simulink model "orthosis_old"  (R2013a)
settings: Solver=FixedStepDiscrete  StartTime=0.0  StopTime=15  FixedStep=.1  RelTol=1e-3
undefined symbols (not defined in the file or in its folder): DiscIntNeverNeededParam
libraries: simulink x7
settings Model: xpc_rtwmakecfg_data=_xpccanac2pci_  BufferReuse=off  Creator=dholley  LastModifiedBy=dholley
settings SolverCC: AlgebraicLoopSolver=LineSearch
settings OptimizationCC: BlockReduction=off  OptimizeBlockIOStorage=off  BufferReuse=off  ExpressionFolding=off  LocalBlockOutputs=off
settings HardwareCC: ProdIntDivRoundTo=Zero  ProdEndianess=LittleEndian  ProdHWDeviceType=Generic->32-bit x86 compatible
settings RTWCC: SystemTargetFile=xpctarget.tlc  TemplateMakefile=xpc_default_tmf  Description=xPC Target  ProcessScript=xpctarget_make_rtw_hook  RTWCompilerOptimization=On
settings xpcTargetCC: TargetFcnLib=ansi_tfl_table_tmw.mat  CodeReplacementLibrary=XPC_BLAS  ParMdlRefBuildCompliant=on  ConcurrentExecutionCompliant=on  CombineSignalStateStructs=off  MATLABClassNameForMDSCustomization=xpcAperiodicCustomization  GRTInterface=on  GenerateAllocFcn=off  xPCTaskExecutionProfile=off  xPCRL32EventNumber=5000  xPCLoadParamSetFile=off  xPCConcurrentTasks=off  xPCEnableSFAnimation=off

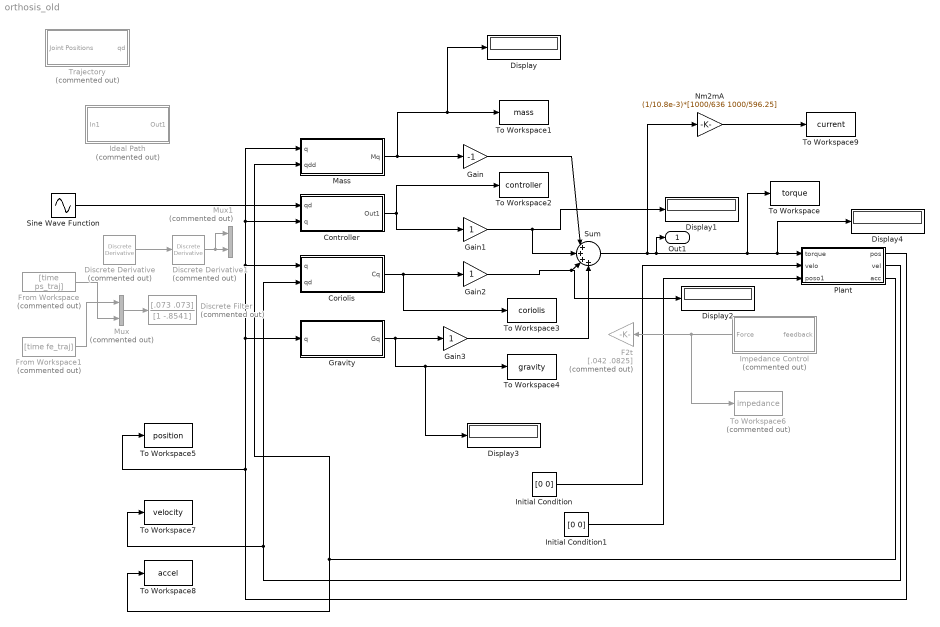
== system orthosis_old ==
  Controller : Subsystem  TreatAsAtomicUnit=on
      settings: RTWSystemCode=Inline
  Coriolis : Subsystem  TreatAsAtomicUnit=on
      settings: RTWSystemCode=Inline
  Discrete Derivative : simulink/Discrete/Discrete Derivative  Commented=on  gainval=1.0  ICPrevScaledInput=0.0  OutMin=[]  OutMax=[]  OutDataType=fixdt(1, 16)  OutScaling=2^-10  DoSatur=off
  Discrete Derivative1 : simulink/Discrete/Discrete Derivative  Commented=on  gainval=1.0  ICPrevScaledInput=0.0  OutMin=[]  OutMax=[]  OutDataType=fixdt(1, 16)  OutScaling=2^-10  DoSatur=off
  Discrete Filter : DiscreteFilter  Commented=on  Numerator=[.073 .073]  Denominator=[1 -.8541]  SampleTime=.001
  Display{,1..4} (5 alike) : Display
  F2t : Gain  Commented=on  Gain=[.042 .0825]
  From Workspace : FromWorkspace  Commented=on  VariableName=[time ps_traj]  SampleTime=0
  From Workspace1 : FromWorkspace  Commented=on  VariableName=[time fe_traj]  SampleTime=0
  Gain : Gain  Gain=-1
  Gain1 : Gain
  Gain2 : Gain
  Gain3 : Gain
  Gravity : Subsystem  TreatAsAtomicUnit=on
      settings: RTWSystemCode=Inline
  Ideal Path : Subsystem  Commented=on
  Impedance Control : Subsystem  Commented=on
  Initial Condition : Constant  Value=[0 0]
  Initial Condition1 : Constant  Value=[0 0]
  Mass : Subsystem  TreatAsAtomicUnit=on
      settings: RTWSystemCode=Inline
  Mux : Mux  Commented=on  Inputs=2
  Mux1 : Mux  Commented=on  Inputs=2
  Nm2mA : Gain  Gain=(1/10.8e-3)*[1000/636 1000/596.25]
  Plant : Subsystem  TreatAsAtomicUnit=on
      settings: MinAlgLoopOccurrences=on  RTWSystemCode=Inline
  Sine Wave Function : Sin  Amplitude=pi/4  Frequency=4
  Sum : Sum  Inputs=|++++
  To Workspace : ToWorkspace  VariableName=torque  SampleTime=-1  SaveFormat=Timeseries
  To Workspace1 : ToWorkspace  VariableName=mass  SampleTime=-1  SaveFormat=Timeseries
  To Workspace2 : ToWorkspace  VariableName=controller  SampleTime=-1  SaveFormat=Timeseries
  To Workspace3 : ToWorkspace  VariableName=coriolis  SampleTime=-1  SaveFormat=Timeseries
  To Workspace4 : ToWorkspace  VariableName=gravity  SampleTime=-1  SaveFormat=Timeseries
  To Workspace5 : ToWorkspace  VariableName=position  SampleTime=-1  SaveFormat=Timeseries
  To Workspace6 : ToWorkspace  Commented=on  VariableName=impedance  SampleTime=-1  SaveFormat=Timeseries
  To Workspace7 : ToWorkspace  VariableName=velocity  SampleTime=-1  SaveFormat=Timeseries
  To Workspace8 : ToWorkspace  VariableName=accel  SampleTime=-1  SaveFormat=Timeseries
  To Workspace9 : ToWorkspace  VariableName=current  SampleTime=-1  SaveFormat=Timeseries
  Trajectory : Subsystem  Commented=on
  Out1 : Outport
  wires:
  Mass/1(Mq) -> Gain/1, Display/1, To Workspace1/1
  Coriolis/1(Cq) -> To Workspace3/1, Gain2/1
  Gravity/1(Gq) -> Gain3/1, Display3/1, To Workspace4/1
  Controller/1(Out1) -> Gain1/1, To Workspace2/1
  Gain3/1 -> Sum/4
  Gain2/1 -> Display2/1, Sum/3
  Gain1/1 -> Display1/1, Sum/2
  Gain/1 -> Sum/1
  Plant/1(pos) -> Gravity/1(q), Controller/2(q), Mass/1(q), Coriolis/1(q), To Workspace5/1
  Initial Condition/1 -> Plant/2(velo)
  Initial Condition1/1 -> Plant/3(poso1)
  Plant/3(acc) -> Mass/2(qdd), To Workspace8/1
  Plant/2(vel) -> Coriolis/2(qd), To Workspace7/1
  Mux/1 -> Discrete Filter/1
  From Workspace/1 -> Mux/2
  From Workspace1/1 -> Mux/1
  Sum/1 -> Nm2mA/1, Out1/1, Display4/1, Plant/1(torque), To Workspace/1
  Sine Wave Function/1 -> Controller/1(qd)
  Impedance Control/1(Force) -> To Workspace6/1, F2t/1
  Discrete Derivative/1 -> Discrete Derivative1/1
  Discrete Derivative1/1 -> Mux1/1, Mux1/2
  Nm2mA/1 -> To Workspace9/1

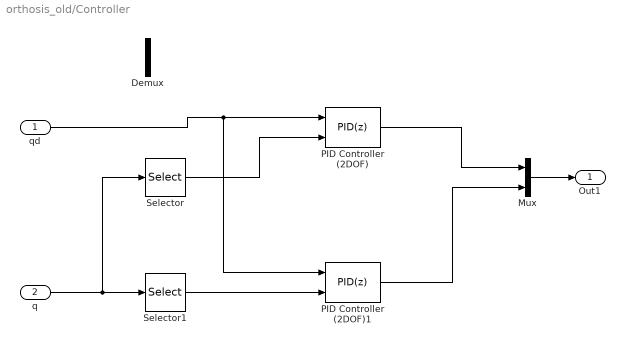
== system orthosis_old/Controller ==
  qd : Inport
  q : Inport  Port=2
  Demux : Demux  Outputs=2
  Mux : Mux  Inputs=2
  PID Controller (2DOF) : simulink/Continuous/PID Controller (2DOF)  Controller=PID  TimeDomain=Discrete-time  SampleTime=-1  IntegratorMethod=Forward Euler  FilterMethod=Forward Euler  Form=Parallel  P=0.000382424241826398  I=3.58199006661761e-06  D=0.00906317872058173  N=18.0350756688688  b=1  c=1  InitialConditionSource=internal  InitialConditionForIntegrator=0  InitialConditionForFilter=0  ExternalReset=none  LimitOutput=off  UpperSaturationLimit=inf  LowerSaturationLimit=-inf  LinearizeAsGain=on  AntiWindupMode=none  Kb=1  TrackingMode=off  Kt=1  PParamMin=[]  PParamMax=[]  IParamMin=[]  IParamMax=[]  DParamMin=[]  DParamMax=[]  NParamMin=[]  NParamMax=[]  bParamMin=[]  bParamMax=[]  cParamMin=[]  cParamMax=[]  KbParamMin=[]  KbParamMax=[]  KtParamMin=[]  KtParamMax=[]  POutMin=[]  POutMax=[]  IOutMin=[]  IOutMax=[]  DOutMin=[]  DOutMax=[]  NOutMin=[]  NOutMax=[]  bOutMin=[]  bOutMax=[]  cOutMin=[]  cOutMax=[]  KbOutMin=[]  KbOutMax=[]  KtOutMin=[]  KtOutMax=[]  IntegratorOutMin=[]  IntegratorOutMax=[]  FilterOutMin=[]  FilterOutMax=[]  SumOutMin=[]  SumOutMax=[]  Sum1OutMin=[]  Sum1OutMax=[]  Sum2OutMin=[]  Sum2OutMax=[]  Sum3OutMin=[]  Sum3OutMax=[]  SumI1OutMin=[]  SumI1OutMax=[]  SumI2OutMin=[]  SumI2OutMax=[]  SumI3OutMin=[]  SumI3OutMax=[]  SumDOutMin=[]  SumDOutMax=[]  SaturationOutMin=[]  SaturationOutMax=[]  IntegratorContinuousStateAttributes=''  IntegratorStateMustResolveToSignalObject=off  IntegratorRTWStateStorageClass=Auto  FilterContinuousStateAttributes=''  FilterStateMustResolveToSignalObject=off  FilterRTWStateStorageClass=Auto
  PID Controller (2DOF)1 : simulink/Continuous/PID Controller (2DOF)  Controller=PID  TimeDomain=Discrete-time  SampleTime=-1  IntegratorMethod=Forward Euler  FilterMethod=Forward Euler  Form=Parallel  P=5  I=10  D=2  N=200  b=1  c=1  InitialConditionSource=internal  InitialConditionForIntegrator=0  InitialConditionForFilter=0  ExternalReset=none  LimitOutput=off  UpperSaturationLimit=inf  LowerSaturationLimit=-inf  LinearizeAsGain=on  AntiWindupMode=none  Kb=1  TrackingMode=off  Kt=1  PParamMin=[]  PParamMax=[]  IParamMin=[]  IParamMax=[]  DParamMin=[]  DParamMax=[]  NParamMin=[]  NParamMax=[]  bParamMin=[]  bParamMax=[]  cParamMin=[]  cParamMax=[]  KbParamMin=[]  KbParamMax=[]  KtParamMin=[]  KtParamMax=[]  POutMin=[]  POutMax=[]  IOutMin=[]  IOutMax=[]  DOutMin=[]  DOutMax=[]  NOutMin=[]  NOutMax=[]  bOutMin=[]  bOutMax=[]  cOutMin=[]  cOutMax=[]  KbOutMin=[]  KbOutMax=[]  KtOutMin=[]  KtOutMax=[]  IntegratorOutMin=[]  IntegratorOutMax=[]  FilterOutMin=[]  FilterOutMax=[]  SumOutMin=[]  SumOutMax=[]  Sum1OutMin=[]  Sum1OutMax=[]  Sum2OutMin=[]  Sum2OutMax=[]  Sum3OutMin=[]  Sum3OutMax=[]  SumI1OutMin=[]  SumI1OutMax=[]  SumI2OutMin=[]  SumI2OutMax=[]  SumI3OutMin=[]  SumI3OutMax=[]  SumDOutMin=[]  SumDOutMax=[]  SaturationOutMin=[]  SaturationOutMax=[]  IntegratorContinuousStateAttributes=''  IntegratorStateMustResolveToSignalObject=off  IntegratorRTWStateStorageClass=Auto  FilterContinuousStateAttributes=''  FilterStateMustResolveToSignalObject=off  FilterRTWStateStorageClass=Auto
  Selector : Selector  InputPortWidth=2  IndexOptions=Index vector (dialog)  Indices=[1]  OutputSizes=1
  Selector1 : Selector  InputPortWidth=2  IndexOptions=Index vector (dialog)  Indices=[2]  OutputSizes=1
  Out1 : Outport
  wires:
  q/1 -> Selector/1, Selector1/1
  Selector/1 -> PID Controller (2DOF)/2
  Selector1/1 -> PID Controller (2DOF)1/2
  Mux/1 -> Out1/1
  qd/1 -> PID Controller (2DOF)1/1, PID Controller (2DOF)/1
  PID Controller (2DOF)/1 -> Mux/1
  PID Controller (2DOF)1/1 -> Mux/2

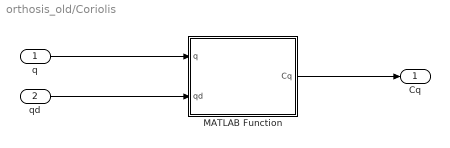
== system orthosis_old/Coriolis ==
  q : Inport
  qd : Inport  Port=2
  MATLAB Function : MATLAB Function  TreatAsAtomicUnit=on
  Cq : Outport
  wires:
  q/1 -> MATLAB Function/1(q)
  MATLAB Function/1(Cq) -> Cq/1
  qd/1 -> MATLAB Function/2(qd)

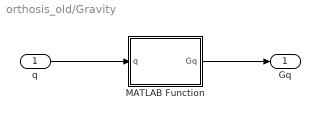
== system orthosis_old/Gravity ==
  q : Inport
  MATLAB Function : MATLAB Function  TreatAsAtomicUnit=on
  Gq : Outport
  wires:
  q/1 -> MATLAB Function/1(q)
  MATLAB Function/1(Gq) -> Gq/1

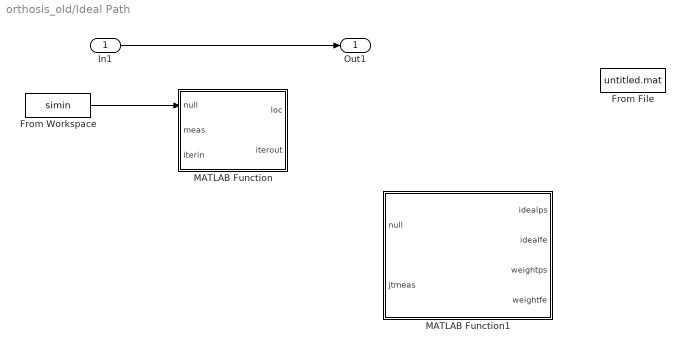
== system orthosis_old/Ideal Path ==
  In1 : Inport
  From Workspace : FromWorkspace  VariableName=simin  SampleTime=0
  From File : FromFile  SampleTime=0
  MATLAB Function : MATLAB Function  TreatAsAtomicUnit=on
  MATLAB Function1 : MATLAB Function  TreatAsAtomicUnit=on
  Out1 : Outport
  wires:
  In1/1 -> Out1/1
  From Workspace/1 -> MATLAB Function/1(null)

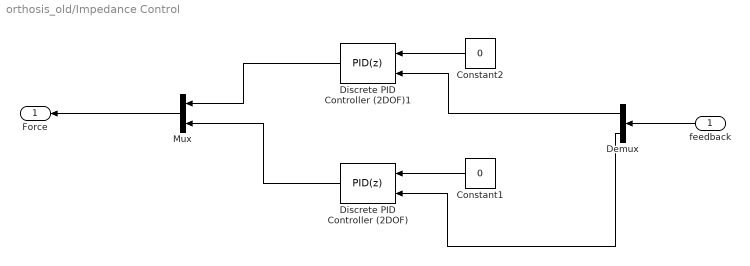
== system orthosis_old/Impedance Control ==
  feedback : Inport
  Constant1 : Constant  Value=0
  Constant2 : Constant  Value=0
  Demux : Demux  Outputs=2
  Discrete PID Controller (2DOF) : simulink/Continuous/PID Controller (2DOF)  Controller=PID  TimeDomain=Discrete-time  SampleTime=.001  IntegratorMethod=Forward Euler  FilterMethod=Forward Euler  Form=Parallel  P=10  I=1  D=0  N=100  b=1  c=1  InitialConditionSource=internal  InitialConditionForIntegrator=0  InitialConditionForFilter=0  ExternalReset=none  LimitOutput=off  UpperSaturationLimit=inf  LowerSaturationLimit=-inf  LinearizeAsGain=off  AntiWindupMode=none  Kb=1  TrackingMode=off  Kt=1  PParamMin=[]  PParamMax=[]  IParamMin=[]  IParamMax=[]  DParamMin=[]  DParamMax=[]  NParamMin=[]  NParamMax=[]  bParamMin=[]  bParamMax=[]  cParamMin=[]  cParamMax=[]  KbParamMin=[]  KbParamMax=[]  KtParamMin=[]  KtParamMax=[]  POutMin=[]  POutMax=[]  IOutMin=[]  IOutMax=[]  DOutMin=[]  DOutMax=[]  NOutMin=[]  NOutMax=[]  bOutMin=[]  bOutMax=[]  cOutMin=[]  cOutMax=[]  KbOutMin=[]  KbOutMax=[]  KtOutMin=[]  KtOutMax=[]  IntegratorOutMin=[]  IntegratorOutMax=[]  FilterOutMin=[]  FilterOutMax=[]  SumOutMin=[]  SumOutMax=[]  Sum1OutMin=[]  Sum1OutMax=[]  Sum2OutMin=[]  Sum2OutMax=[]  Sum3OutMin=[]  Sum3OutMax=[]  SumI1OutMin=[]  SumI1OutMax=[]  SumI2OutMin=[]  SumI2OutMax=[]  SumI3OutMin=[]  SumI3OutMax=[]  SumDOutMin=[]  SumDOutMax=[]  SaturationOutMin=[]  SaturationOutMax=[]  IntegratorContinuousStateAttributes=''  IntegratorStateMustResolveToSignalObject=off  IntegratorRTWStateStorageClass=Auto  FilterContinuousStateAttributes=''  FilterStateMustResolveToSignalObject=off  FilterRTWStateStorageClass=Auto
  Discrete PID Controller (2DOF)1 : simulink/Continuous/PID Controller (2DOF)  Controller=PID  TimeDomain=Discrete-time  SampleTime=.001  IntegratorMethod=Forward Euler  FilterMethod=Forward Euler  Form=Parallel  P=10  I=10  D=0  N=100  b=1  c=1  InitialConditionSource=internal  InitialConditionForIntegrator=0  InitialConditionForFilter=0  ExternalReset=none  LimitOutput=off  UpperSaturationLimit=inf  LowerSaturationLimit=-inf  LinearizeAsGain=off  AntiWindupMode=none  Kb=1  TrackingMode=off  Kt=1  PParamMin=[]  PParamMax=[]  IParamMin=[]  IParamMax=[]  DParamMin=[]  DParamMax=[]  NParamMin=[]  NParamMax=[]  bParamMin=[]  bParamMax=[]  cParamMin=[]  cParamMax=[]  KbParamMin=[]  KbParamMax=[]  KtParamMin=[]  KtParamMax=[]  POutMin=[]  POutMax=[]  IOutMin=[]  IOutMax=[]  DOutMin=[]  DOutMax=[]  NOutMin=[]  NOutMax=[]  bOutMin=[]  bOutMax=[]  cOutMin=[]  cOutMax=[]  KbOutMin=[]  KbOutMax=[]  KtOutMin=[]  KtOutMax=[]  IntegratorOutMin=[]  IntegratorOutMax=[]  FilterOutMin=[]  FilterOutMax=[]  SumOutMin=[]  SumOutMax=[]  Sum1OutMin=[]  Sum1OutMax=[]  Sum2OutMin=[]  Sum2OutMax=[]  Sum3OutMin=[]  Sum3OutMax=[]  SumI1OutMin=[]  SumI1OutMax=[]  SumI2OutMin=[]  SumI2OutMax=[]  SumI3OutMin=[]  SumI3OutMax=[]  SumDOutMin=[]  SumDOutMax=[]  SaturationOutMin=[]  SaturationOutMax=[]  IntegratorContinuousStateAttributes=''  IntegratorStateMustResolveToSignalObject=off  IntegratorRTWStateStorageClass=Auto  FilterContinuousStateAttributes=''  FilterStateMustResolveToSignalObject=off  FilterRTWStateStorageClass=Auto
  Mux : Mux  Inputs=2
  Force : Outport
  wires:
  Constant1/1 -> Discrete PID Controller (2DOF)/1
  Constant2/1 -> Discrete PID Controller (2DOF)1/1
  Discrete PID Controller (2DOF)1/1 -> Mux/1
  Discrete PID Controller (2DOF)/1 -> Mux/2
  Mux/1 -> Force/1
  feedback/1 -> Demux/1
  Demux/2 -> Discrete PID Controller (2DOF)/2
  Demux/1 -> Discrete PID Controller (2DOF)1/2

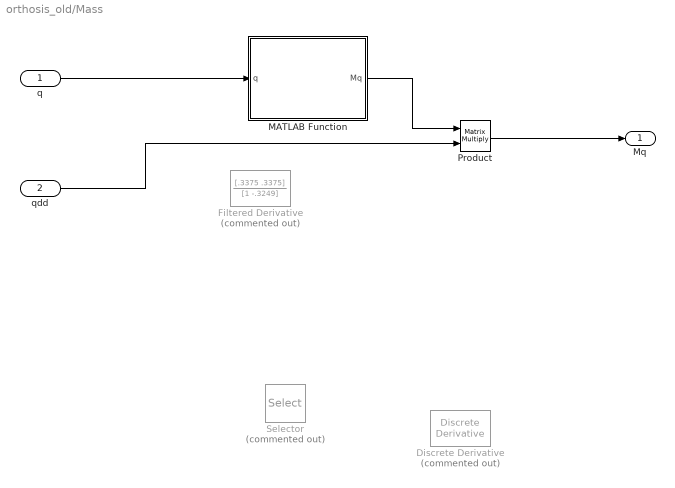
== system orthosis_old/Mass ==
  q : Inport
  qdd : Inport  Port=2
  Discrete Derivative : simulink/Discrete/Discrete Derivative  Commented=on  gainval=.1  ICPrevScaledInput=0.0  OutMin=[]  OutMax=[]  OutDataType=fixdt(1, 16)  OutScaling=2^-10  DoSatur=off
  Filtered Derivative : DiscreteFilter  Commented=on  Numerator=[.3375 .3375]  Denominator=[1 -.3249]  SampleTime=.1
  MATLAB Function : MATLAB Function  TreatAsAtomicUnit=on
  Product : Product  Multiplication=Matrix(*)  RndMeth=Zero
  Selector : Selector  Commented=on  InputPortWidth=4  IndexOptions=Index vector (dialog)  Indices=[3:4]  OutputSizes=1
  Mq : Outport
  wires:
  q/1 -> MATLAB Function/1(q)
  MATLAB Function/1(Mq) -> Product/1
  Product/1 -> Mq/1
  qdd/1 -> Product/2

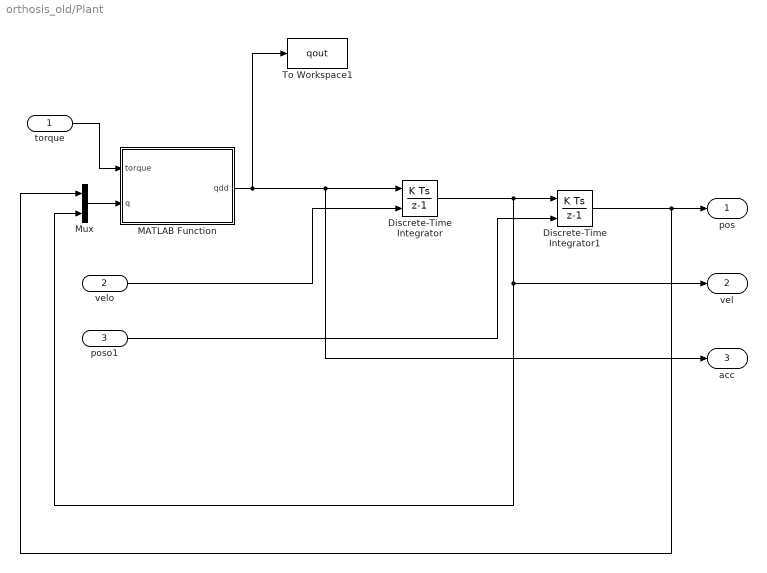
== system orthosis_old/Plant ==
  torque : Inport
  velo : Inport  Port=2
  poso1 : Inport  Port=3
  Discrete-Time Integrator : DiscreteIntegrator  gainval=1  InitialConditionSource=external  SampleTime=-1  ICPrevOutput=DiscIntNeverNeededParam  ICPrevScaledInput=DiscIntNeverNeededParam
  Discrete-Time Integrator1 : DiscreteIntegrator  gainval=1  InitialConditionSource=external  SampleTime=-1  ICPrevOutput=DiscIntNeverNeededParam  ICPrevScaledInput=DiscIntNeverNeededParam
  MATLAB Function : MATLAB Function  TreatAsAtomicUnit=on
  Mux : Mux  Inputs=2
  To Workspace1 : ToWorkspace  VariableName=qout  SampleTime=-1  SaveFormat=Timeseries
  pos : Outport
  vel : Outport  Port=2
  acc : Outport  Port=3
  wires:
  torque/1 -> MATLAB Function/1(torque)
  MATLAB Function/1(qdd) -> acc/1, Discrete-Time Integrator/1, To Workspace1/1
  velo/1 -> Discrete-Time Integrator/2
  Discrete-Time Integrator1/1 -> Mux/1, pos/1
  Discrete-Time Integrator/1 -> vel/1, Mux/2, Discrete-Time Integrator1/1
  poso1/1 -> Discrete-Time Integrator1/2
  Mux/1 -> MATLAB Function/2(q)

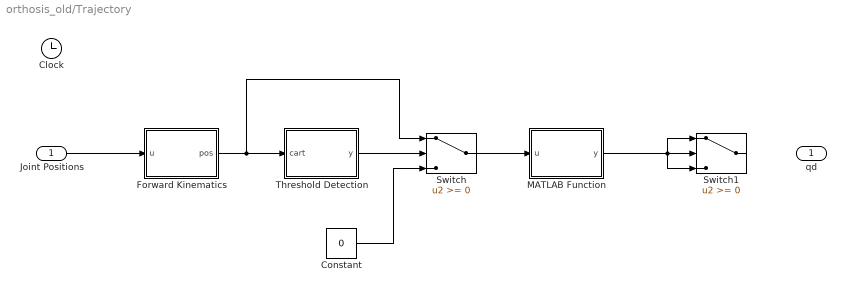
== system orthosis_old/Trajectory ==
  Joint Positions : Inport
  Clock : Clock
  Constant : Constant  Value=0
  Forward Kinematics : MATLAB Function  TreatAsAtomicUnit=on
  MATLAB Function : MATLAB Function  TreatAsAtomicUnit=on
  Switch : Switch
  Switch1 : Switch
  Threshold Detection : MATLAB Function  TreatAsAtomicUnit=on
  qd : Outport
  wires:
  Joint Positions/1 -> Forward Kinematics/1(u)
  Forward Kinematics/1(pos) -> Switch/1, Threshold Detection/1(cart)
  Threshold Detection/1(y) -> Switch/2
  Constant/1 -> Switch/3
  Switch/1 -> MATLAB Function/1(u)
  MATLAB Function/1(y) -> Switch1/3, Switch1/1, Switch1/2

== matlab function orthosis_old/Coriolis/MATLAB Function ==
  data: q input; Cq output; qd input
function Cq = Coriolis(q,qd)
%#codegen

weight=(85.4');%kg
hand_length=(.189);%m
hand_width=(.084);%m

s7=sin(q(2));
c7=cos(q(2));
a7cm=-.00458;
d7cm=-.00285;
a6=.03952;
m7=.2256; %kg

hand_xcom=0;
hand_ycom=-hand_length*.468;
hand_zcom=hand_width/2;
hand_mass=weight*.00575;

com7=[a7cm;-.03363;d7cm]*m7 + [hand_xcom;hand_ycom;hand_zcom]*hand_mass/(m7 + hand_mass);

%Centrifugal
c112=-m7*com7(1)^2*s7*c7;
C1C2=[0 0;c112 0];

%Coriolis
c121=-m7*com7(1)^2*s7*c7;
c122=m7*com7(1)*com7(3)*c7;
C22=[c121;c122];

Cq=C22*(qd(1)*qd(2)) + C1C2*[qd(1)^2;qd(2)^2];

== matlab function orthosis_old/Mass/MATLAB Function ==
  data: q input; Mq output
function Mq  = massmatrix(q)

%%Input Metrics
height=(1.776);%m
weight=(85.4);%kg
hand_length=(.189);%m
hand_width=(.084);%m
hand_thick=(.028);%m

% s1=sind(q(1));
% c1=cosd(q(1));
% s2=sind(q(2));
% c2=cosd(q(2));
% s4=sind(q(4));
% c4=cosd(q(4));
% s5=sind(q(5));
% c5=cosd(q(5));
s6=sin(q(1));
c6=cos(q(1));
s7=sin(q(2));
c7=cos(q(2));

m6=.4242; %kg
m7=.2256; %kg

%in m
a6cm=.02382;
d6cm=.04397;
a7cm=-.00458;
d7cm=-.00285;
d6=.06708;
a6=.03952;
a5=.12051;
d4=.04586;
a2=.37546;
d1=.33655;

%Forearm Inertia
forearm_length=height*.1585;
forearm_mass=weight*.016;
forearm_volume=forearm_mass/1062;
forearm_radius=sqrt(forearm_volume/(pi*forearm_length));

arm_zcom=d6-(forearm_length*.568);
arm_xcom=a6-forearm_radius;
arm_ycom=0;


kx_forearm=forearm_radius*.276;
ky_forearm=forearm_radius*.265;
kz_forearm=forearm_length*.121;
Ixx_forearm=forearm_mass*kx_forearm^2 + forearm_mass*arm_zcom^2;
Iyy_forearm=forearm_mass*ky_forearm^2 + forearm_mass*(arm_xcom^2 + arm_zcom^2);
Izz_forearm=forearm_mass*kz_forearm^2 + forearm_mass*arm_xcom^2;
Ixy_forearm=0;
Ixz_forearm=forearm_mass*arm_xcom*arm_zcom;
Iyz_forearm=0;

I_forearm=[Ixx_forearm,-Ixy_forearm,-Ixz_forearm;-Ixy_forearm,Iyy_forearm,-Iyz_forearm;-Ixz_forearm,-Iyz_forearm,Izz_forearm];

%Hand Inertia
hand_xcom=0;
hand_ycom=-hand_length*.468;
hand_zcom=hand_width/2;
hand_mass=weight*.00575;

kx_hand=hand_thick*.235;
ky_hand=hand_length*.184;
kz_hand=hand_width*.288;
Ixx_hand=hand_mass*kx_hand^2 + hand_mass*(hand_ycom^2 + hand_zcom^2);
Iyy_hand=hand_mass*ky_hand^2 + hand_mass*hand_zcom^2;
Izz_hand=hand_mass*kz_hand^2 + hand_mass*hand_ycom^2;
Ixy_hand=0;
Ixz_hand=0;
Iyz_hand=hand_mass*hand_ycom*hand_zcom;

I_hand=[Ixx_hand,-Ixy_hand,-Ixz_hand;-Ixy_hand,Iyy_hand,-Iyz_hand;-Ixz_hand,-Iyz_hand,Izz_hand];


I6=[2.259e-3 -7.049e-5 -9.252e-5;-7.049e-5 2.091e-3 -4.603e-4;-9.252e-5 -4.603e-4 8.911e-4];
I7=[7.022e-4 8.207e-5 -2.535e-5;8.207e-5 1.675e-4 -1.046e-4;-2.535e-5 -1.046e-4 6.273e-4];

%Forward Kinematics for Positioning
% x=-a5*c1*s2*c5 - a5*s5*(s1*c4 - c1*c2*s4) - d4*c1*s2 + d3*c1*c2 + a2*c1*c2;
% y=-a5*s1*s2*c5 + a5*s5*(c1*c4 + s1*c2*c4) - d4*s1*s2 + d3*s1*c2 + a2*s1*c2;
% z=-a5*c2*c5 - a5*s2*s4*s5 - d4*c2 - d3*s2 - a2*s2 + d1;

%Modified Center of Mass Location
com6=[a6cm;-.01547;d6cm]*m6 + [arm_xcom;arm_ycom;arm_zcom]*forearm_mass/(m6 + forearm_mass);
com7=[a7cm;-.03363;d7cm]*m7 + [hand_xcom;hand_ycom;hand_zcom]*hand_mass/(m7 + hand_mass);

%Jacobian
Jv1=[-com6(1)*s6,0;com6(1)*c6,0;0,0];
Jv2=[-com7(1)*c6*c7 + com7(3)*s6 - a6*c6,com7(1)*s6*s7;-com7(1)*s6*c7 - com7(3)*c6 - a6*s6,-com7(1)*c6*s7;0,-com7(1)*c7];

Jw1=[0,0;0,0;1,0];
Jw2=[0,-c6;0,-s6;1,0];

%Rotation Matrix
R6=[-s6,0,-c6;c6,0,-s6;0,-1,0];

D6=m6*(Jv1'*Jv1)+Jw1'*(I6 + I_forearm)*Jw1;
D7=m7*(Jv2'*Jv2)+Jw2'*R6*(I7 + I_hand)*R6'*Jw2;
D=D6+D7;%Mass Matrix

Mq=D;

== matlab function orthosis_old/Gravity/MATLAB Function ==
  data: q input; Gq output
function Gq = Gravity(q)
%#codegen

height=(1.776);%m
weight=(85.4);%kg
hand_length=(.189);%m
hand_width=(.084);%m

s6=sin(q(1));
c6=cos(q(1));
s7=sin(q(2));
c7=cos(q(2));

m6=.4242; %kg
m7=.2256; %kg

a7cm=-.00458;
d7cm=-.00285;
a6=.03952;
d6=.06708;
a6cm=.01425;
d6cm=.04397;

forearm_length=height*.1585;
forearm_mass=weight*.016;
forearm_volume=forearm_mass/1062;
forearm_radius=sqrt(forearm_volume/(pi*forearm_length));
arm_zcom=d6-(forearm_length*.568);
arm_xcom=a6-forearm_radius;
arm_ycom=0;

hand_xcom=0;
hand_ycom=-hand_length*.468;
hand_zcom=hand_width/2;
hand_mass=weight*.00575;

com6=[a6cm;-.01547;d6cm]*m6 + [arm_xcom;arm_ycom;arm_zcom]*forearm_mass/(m6 + forearm_mass);
com7=[a7cm;-.03363;d7cm]*m7 + [hand_xcom;hand_ycom;hand_zcom]*hand_mass/(m7 + hand_mass);

%Jacobian
Jv1=[-com6(1)*s6,0;com6(1)*c6,0;0,0];
Jv2=[-com7(1)*c6*c7 + com7(3)*s6 - a6*s6,com7(1)*s6*s7;-com7(1)*s6*c7 - com7(3)*c6 + a6*c6,-com7(1)*c6*s7;0,-com7(1)*c7];

Gq=-((Jv1'*m6*[9.81;0;0]) + (Jv2'*m7*[0;0;-9.81]));

== matlab function orthosis_old/Plant/MATLAB Function ==
  data: torque input; qdd output; q input
function qdd  = plantv2(torque,q)

%Forward Kinematics for Positioning
% x=-a5*c1*s2*c5 - a5*s5*(s1*c4 - c1*c2*s4) - d4*c1*s2 + d3*c1*c2 + a2*c1*c2;
% y=-a5*s1*s2*c5 + a5*s5*(c1*c4 + s1*c2*c4) - d4*s1*s2 + d3*s1*c2 + a2*s1*c2;
% z=-a5*c2*c5 - a5*s2*s4*s5 - d4*c2 - d3*s2 - a2*s2 + d1;

% s1=sind(q(1));
% c1=cosd(q(1));
% s2=sind(q(2));
% c2=cosd(q(2));
% s4=sind(q(4));
% c4=cosd(q(4));
% s5=sind(q(5));
% c5=cosd(q(5));
s6=sin(q(1));
c6=cos(q(1));
s7=sin(q(2));
c7=cos(q(2));

m6=.4242; %kg
m7=.2256; %kg

I6=[2.259e-3 -7.049e-5 -9.252e-5;-7.049e-5 2.091e-3 -4.603e-4;-9.252e-5 -4.603e-4 8.911e-4];
I7=[7.022e-4 8.207e-5 -2.535e-5;8.207e-5 1.675e-4 -1.046e-4;-2.535e-5 -1.046e-4 6.273e-4];

%in m
a6cm=.01425;
d6cm=.01386;
a7cm=-.00458;
d7cm=-.00285;
a6=.03952;
a5=.12051;
d4=.04586;
a2=.37546;
d1=.33655;

%Jacobian
Jv1=[-a6cm*s6,0;a6cm*c6,0;0,0];
Jv2=[-a7cm*c6*c7 + d7cm*s6 - a6*c6,a7cm*s6*s7;-a7cm*s6*c7 - d7cm*c6 - a6*s6,-a7cm*c6*s7;0,-a7cm*c7];

Jw1=[0,0;0,0;1,0];
Jw2=[0,-c6;0,-s6;1,0];

%Rotation Matrix
R6=[-s6,0,-c6;c6,0,-s6;0,-1,0];

D6=m6*(Jv1'*Jv1)+Jw1'*I6*Jw1;
D7=m7*(Jv2'*Jv2)+Jw2'*R6*I7*R6'*Jw2;
D=D6+D7;%Mass Matrix

%Centrifugal
c112=-m7*a7cm^2*s7*c7;
C1C2=[0 0;c112 0];

%Coriolis
c121=-m7*a7cm^2*s7*c7;
c122=m7*a7cm*d7cm*c7;
C22=[c121;c122];

Cq=C22*(q(3)*q(4)) + C1C2*[q(3)^2;q(4)^2];

%Gravitational
G=-((Jv1'*m6*[9.81;0;0]) + (Jv2'*m7*[0;0;-9.81]));

% Dcond=[eye(2),zeros(2);zeros(2),-D];
% qdd=Dcond\[q(3:4);(Cq+G-torque)];

qdd=-D\(Cq+G-torque);

== matlab function orthosis_old/Trajectory/Forward Kinematics ==
  data: u input; pos output

function pos = fkin(u)

s1=sind(u(1));
c1=cosd(u(1));
s2=sind(u(2));
c2=cosd(u(2));
s4=sind(u(4));
c4=cosd(u(4));
s5=sind(u(5));
c5=cosd(u(5));
s6=sind(u(6));
c6=cosd(u(6));

a6=.03952;
d6=.06708;
a5=.12051;
d4=.04586;
d3=u(3);
a2=.37546;
d1=.33655;

%Forward Kinematics for Positioning
x=-a6*c6*(c1*s2*c5 + s5*(s1*c4 - c1*c2*s4)) + a6*s6*(s1*s4 + c1*c2*c4) - d6*(c1*s2*s5 - c5*(s1*c4 - c1*c2*s4)) - a5*c1*s2*c5 - a5*s5*(s1*c4 - c1*c2*s4) - d4*c1*s2 + d3*c1*c2 + a2*c1*c2;
y=-a6*c6*(s1*s2*c5 - s5*(c1*c4 + s1*c2*s4)) - a6*s6*(c1*s4 - s1*c2*c4) - d6*(s1*s2*s5 + c5*(c1*c4 + s1*c2*s4)) - a5*s1*s2*c5 + a5*s5*(c1*c4 + s1*c2*c4) - d4*s1*s2 + d3*s1*c2 + a2*s1*c2;
z=-a6*c6*(c2*c5 + s2*s4*s5) - a6*s2*c4*s6 - d6*(c2*s5 - s2*s4*c5) - a5*c2*c5 - a5*s2*s4*s5 - d4*c2 - d3*s2 - a2*s2 + d1;

pos=[x;y;z];

== matlab function orthosis_old/Trajectory/Threshold Detection ==
  data: cart input; y output
function y = thres(cart)
% function y = thres(cart)
% 
% %Object Position
% xo=
% yo=
% zo=
% 
% %Orthosis Position
% xw=cart(1);
% yw=cart(2);
% zw=cart(3);
% 
% delta_r=abs(sqrt((xw-xo)^2 + (yw-yo)^2 + (zw-zo)^2));
% 
% threshold=
%     
% y = threshold - delta_r;

== matlab function orthosis_old/Trajectory/MATLAB Function ==
  data: u input; y output
%%Approach Angle Measurement and Trajectory Selection

function y = fcn(u)
%#codegen

%if u(1)> 0 & u(2)>0 & u(3)>0
%   calculate approach angle
%   measured in x-y plane relative to x-axis
%   select trajectory based on approach zone

%else
%   quit
y = u;

== matlab function orthosis_old/Ideal Path/MATLAB Function ==
  data: null input; loc output; meas input; iterin input; iterout output
function [loc,iterout] = position(null,meas,iterin)
%#codegen


% 
% for i=1:1000
%     if meas(1)<=null(2,i) && meas(1)>=null(3,i) && meas(2)<=null(5,i) && meas(2)>=null(6,i) && meas(3)<=null(8,i) && meas(3)>=null(9,i)
%         loc(n)=i;
%         dist(n)=sqrt((meas(1)-null(1,i))^2 + (meas(2)-null(4,i))^2 + (meas(3)-null(7,i))^2);
%         n=n+1;
%     else
%         continue
%     end
% end

while iterin < 160
    dist=zeros(1,160);
    for i=1:160
        dist(i)=sqrt((meas(1)-null(1,i))^2 + (meas(2)-null(4,i))^2 + (meas(3)-null(7,i))^2);
    end
    [~,iter]=min(dist);
    loc=[null(1,iter),null(4,iter),null(7,iter),null(10,iter),null(13,iter)];
    iterout=iter;
end

while iterin < 398
    dist=zeros(1,237);
    n=1;
    for i=161:398
        dist(n)=sqrt((meas(1)-null(1,i))^2 + (meas(2)-null(4,i))^2 + (meas(3)-null(7,i))^2);
        n=n+1;
    end
    [~,iter]=min(dist);
    loc=[null(1,iter),null(4,iter),null(7,iter),null(10,iter),null(13,iter)];
    iterout=iter;
end

while iterin < 750
    dist=zeros(1,351);
    n=1;
    for i=1:160
        dist(i)=sqrt((meas(1)-null(1,i))^2 + (meas(2)-null(4,i))^2 + (meas(3)-null(7,i))^2);
        n=n+1;
    end
    [~,iter]=min(dist);
    loc=[null(1,iter),null(4,iter),null(7,iter),null(10,iter),null(13,iter)];
    iterout=iter;
end

while iterin <= 1000
    dist=zeros(1,250);
    n=1;
    for i=1:160
        dist(i)=sqrt((meas(1)-null(1,i))^2 + (meas(2)-null(4,i))^2 + (meas(3)-null(7,i))^2);
        n=n+1;
    end
    [~,iter]=min(dist);
    loc=[null(1,iter),null(4,iter),null(7,iter),null(10,iter),null(13,iter)];
    iterout=iter;
end

if iterin >= 1000
    iterout=0;
end

== matlab function orthosis_old/Ideal Path/MATLAB Function1 ==
  data: idealps output; null input; jtmeas input; idealfe output; weightps output; weightfe output
function [idealps,idealfe,weightps,weightfe] = jtselect(null,jtmeas)
%#codegen

idealps=null(10,cycle);
idealfe=null(13,cycle);

weightps=1./(1+exp((10/(null(10,cycle)-null(11,cycle)))*jtmeas(1)-((null(10,cycle)+null(11,cycle))/2)*(10/(null(10,cycle)-null(11,cycle))))) + 1./(1+exp((10/(null(10,cycle)-null(12,cycle)))*jtmeas(1)-((null(10,cycle)+null(12,cycle))/2)*(10/(null(10,cycle)-null(12,cycle)))));
weightfe=1./(1+exp((10/(null(13,cycle)-null(14,cycle)))*jtmeas(2)-((null(13,cycle)+null(14,cycle))/2)*(10/(null(13,cycle)-null(14,cycle))))) + 1./(1+exp((10/(null(13,cycle)-null(15,cycle)))*jtmeas(2)-((null(13,cycle)+null(15,cycle))/2)*(10/(null(13,cycle)-null(15,cycle)))));

end
